simulink model "ex5_RL"  (R2023a)
settings: Solver=VariableStepAuto  StartTime=0.0  StopTime=30  RelTol=1e-3
values from neighbouring files (symbols this model uses):
  k1 = 5    [ex3_4.m]    (also in ex5.m = 1)
  k2 = 5    [ex3_4.m]    (also in ex5.m = 2.5)
  k3 = 3    [ex5.m]
  theta_i = qi(3)    [ex3_4.m]    (also in ex5.m = 0.785398163397)
  Ts = Ts * scaling    [ex3_4.m]    (also in ex5.m = 0.001)
  x_i = qi(1)    [ex3_4.m]    (also in ex5.m = 10)
  y_i = qi(2)    [ex3_4.m]    (also in ex5.m = 1)
libraries: robotmobilelib x1
settings Model: Creator=Francesco  LastModifiedBy=salvatoregranata
settings DataIOCC: ExternalInput=k1,k2 ,3
settings OptimizationCC: ReuseModelBlockBuffer=off
settings HardwareCC: ProdBitPerLong=64  ProdHWDeviceType=Intel->x86-64 (Mac OS X)

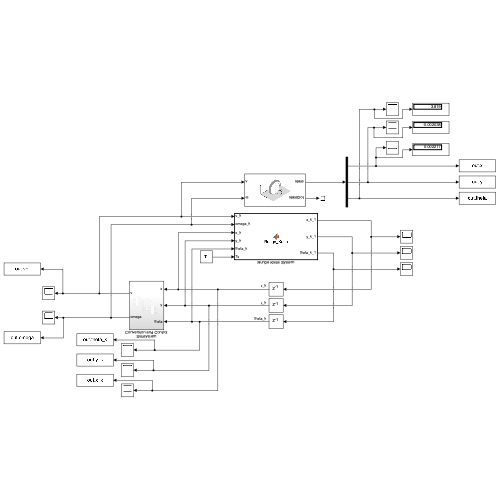
[thumbnail: Simulink's stored preview of the top-level diagram]
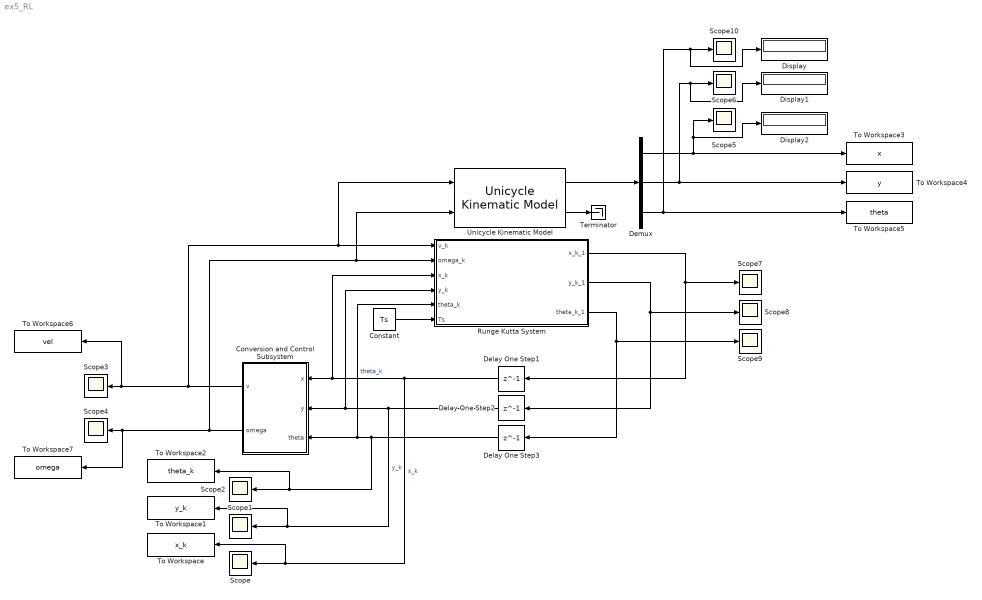
== system ex5_RL ==
  Constant : Constant  Value=Ts
  Conversion and Control Subsystem : Subsystem
  Delay One Step1 : Delay  DelayLength=1  InitialCondition=x_i  SampleTime=Ts
  Delay One Step2 : Delay  DelayLength=1  InitialCondition=y_i  SampleTime=Ts
  Delay One Step3 : Delay  DelayLength=1  InitialCondition=theta_i  SampleTime=Ts
  Demux : Demux  Outputs=3
  Display : Display
  Display1 : Display
  Display2 : Display
  Runge Kutta System : MATLAB Function  TreatAsAtomicUnit=on
  Scope{,1..10} (11 alike) : Scope
  Terminator : Terminator
  To Workspace : ToWorkspace  VariableName=x_k  SampleTime=-1
  To Workspace1 : ToWorkspace  VariableName=y_k  SampleTime=-1
  To Workspace2 : ToWorkspace  VariableName=theta_k  SampleTime=-1
  To Workspace3 : ToWorkspace  VariableName=x  SampleTime=-1
  To Workspace4 : ToWorkspace  VariableName=y  SampleTime=-1
  To Workspace5 : ToWorkspace  VariableName=theta  SaveFormat=Timeseries  SampleTime=-1
  To Workspace6 : ToWorkspace  VariableName=vel  SaveFormat=Timeseries  SampleTime=-1
  To Workspace7 : ToWorkspace  VariableName=omega  SaveFormat=Timeseries  SampleTime=-1
  Unicycle Kinematic Model : robotmobilelib/Unicycle Kinematic Model  VehicleInputs=Vehicle Speed & Heading Angular Velocity  WheelRadius=0.1  WheelSpeedRange=[-Inf Inf]  InitialState=[x_i; y_i; theta_i]  SimulateUsing=Interpreted execution
  wires:
  Runge Kutta System/3(theta_k_1) -> Delay One Step3/1, Scope9/1
  Delay One Step1/1 -> Runge Kutta System/3(x_k), Conversion and Control Subsystem/1(x), To Workspace/1, Scope/1  "x_k"
  Runge Kutta System/1(x_k_1) -> Scope7/1, Delay One Step1/1
  Delay One Step2/1 -> Runge Kutta System/4(y_k), Conversion and Control Subsystem/2(y), To Workspace1/1, Scope1/1  "y_k"
  Runge Kutta System/2(y_k_1) -> Delay One Step2/1, Scope8/1
  Unicycle Kinematic Model/1 -> Demux/1
  Demux/1 -> To Workspace3/1, Scope5/1, Display2/1
  Demux/2 -> To Workspace4/1, Display1/1, Scope6/1
  Delay One Step3/1 -> Conversion and Control Subsystem/3(theta), Runge Kutta System/5(theta_k), Scope2/1, To Workspace2/1  "theta_k"
  Conversion and Control Subsystem/1(v) -> Unicycle Kinematic Model/1, Runge Kutta System/1(v_k), To Workspace6/1, Scope3/1
  Conversion and Control Subsystem/2(omega) -> Unicycle Kinematic Model/2, Runge Kutta System/2(omega_k), To Workspace7/1, Scope4/1
  Demux/3 -> To Workspace5/1, Display/1, Scope10/1
  Unicycle Kinematic Model/2 -> Terminator/1
  Constant/1 -> Runge Kutta System/6(Ts)

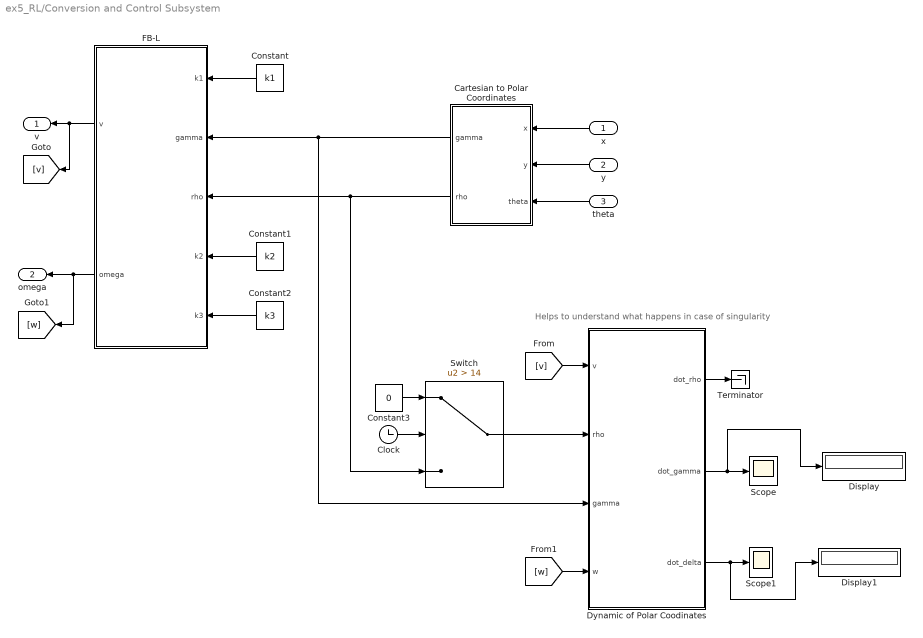
== system ex5_RL/Conversion and Control Subsystem ==
  note: Helps to understand what happens in case of singularity
  x : Inport
  y : Inport  Port=2
  theta : Inport  Port=3
  "Cartesian to Polar Coordinates " : Subsystem
  Clock : Clock
  Constant : Constant  Value=k1
  Constant1 : Constant  Value=k2
  Constant2 : Constant  Value=k3
  Constant3 : Constant  Value=0
  Display : Display
  Display1 : Display
  Dynamic of Polar Coodinates : MATLAB Function  TreatAsAtomicUnit=on
  FB-L : Subsystem
  Scope : Scope
  Scope1 : Scope
  Switch : Switch  Criteria=u2 > Threshold  Threshold=14  SaturateOnIntegerOverflow=off  InputSameDT=off
  Terminator : Terminator
  v : Outport
  omega : Outport  Port=2
  wires:
  Constant/1 -> FB-L/1(k1)
  Constant1/1 -> FB-L/4(k2)
  Constant2/1 -> FB-L/5(k3)
  FB-L/1(v) -> [v], v/1
  FB-L/2(omega) -> [w], omega/1
  x/1 -> "Cartesian to Polar Coordinates "/1(x)
  y/1 -> "Cartesian to Polar Coordinates "/2(y)
  theta/1 -> "Cartesian to Polar Coordinates "/3(theta)
  "Cartesian to Polar Coordinates "/2(rho) -> Switch/3, FB-L/3(rho)
  [v] -> Dynamic of Polar Coodinates/1(v)
  "Cartesian to Polar Coordinates "/1(gamma) -> Dynamic of Polar Coodinates/3(gamma), FB-L/2(gamma)
  [w] -> Dynamic of Polar Coodinates/4(w)
  Dynamic of Polar Coodinates/1(dot_rho) -> Terminator/1
  Dynamic of Polar Coodinates/2(dot_gamma) -> Display/1, Scope/1
  Dynamic of Polar Coodinates/3(dot_delta) -> Display1/1, Scope1/1
  Switch/1 -> Dynamic of Polar Coodinates/2(rho)
  Constant3/1 -> Switch/1
  Clock/1 -> Switch/2

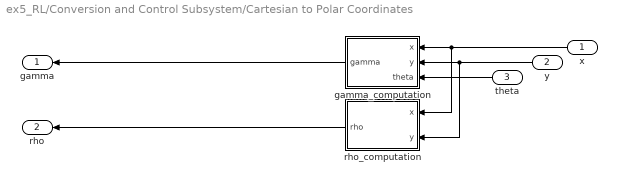
== system ex5_RL/Conversion and Control Subsystem/Cartesian to Polar Coordinates  ==
  x : Inport
  y : Inport  Port=2
  theta : Inport  Port=3
  gamma_computation : MATLAB Function  TreatAsAtomicUnit=on
  rho_computation : MATLAB Function  TreatAsAtomicUnit=on
  gamma : Outport
  rho : Outport  Port=2
  wires:
  gamma_computation/1(gamma) -> gamma/1
  theta/1 -> gamma_computation/3(theta)
  y/1 -> gamma_computation/2(y), rho_computation/2(y)
  rho_computation/1(rho) -> rho/1
  x/1 -> rho_computation/1(x), gamma_computation/1(x)

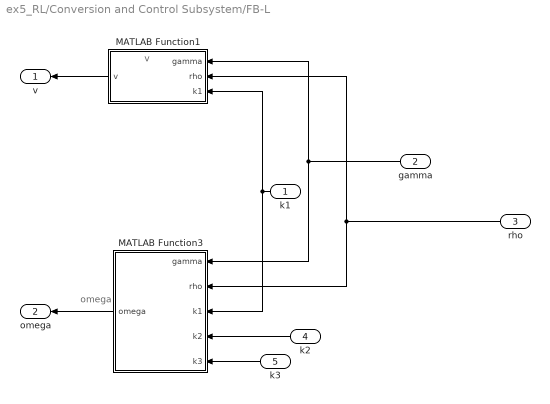
== system ex5_RL/Conversion and Control Subsystem/FB-L ==
  note: omega
  note: v
  k1 : Inport
  gamma : Inport  Port=2
  rho : Inport  Port=3
  k2 : Inport  Port=4
  k3 : Inport  Port=5
  MATLAB Function1 : MATLAB Function  TreatAsAtomicUnit=on
  MATLAB Function3 : MATLAB Function  TreatAsAtomicUnit=on
  v : Outport
  omega : Outport  Port=2
  wires:
  MATLAB Function1/1(v) -> v/1
  MATLAB Function3/1(omega) -> omega/1
  gamma/1 -> MATLAB Function1/1(gamma), MATLAB Function3/1(gamma)
  k1/1 -> MATLAB Function3/3(k1), MATLAB Function1/3(k1)
  k3/1 -> MATLAB Function3/5(k3)
  k2/1 -> MATLAB Function3/4(k2)
  rho/1 -> MATLAB Function3/2(rho), MATLAB Function1/2(rho)

== matlab function ex5_RL/Runge Kutta System ==
  data: v_k input; x_k_1 output; omega_k input; x_k input; y_k_1 output; y_k input; theta_k input; theta_k_1 output; Ts input
function [x_k_1,y_k_1,theta_k_1] = Runge_Kutta(v_k,omega_k,x_k,y_k,theta_k,Ts)

%2nd order Runge-Kutta approximation
x_k_1=x_k+v_k*Ts*cos(theta_k+Ts*omega_k/2);
y_k_1=y_k+v_k*Ts*sin(theta_k+Ts*omega_k/2);
theta_k_1=theta_k+omega_k*Ts;

== matlab function ex5_RL/Conversion and Control Subsystem/Cartesian to Polar Coordinates /rho_computation ==
  data: x input; rho output; y input
function rho = fcn(x,y)

rho=sqrt(x^2 + y^2);

== matlab function ex5_RL/Conversion and Control Subsystem/Cartesian to Polar Coordinates /gamma_computation ==
  data: x input; gamma output; y input; theta input
function gamma = fcn(x,y,theta)
gamma=atan2(y,x)-theta+pi;

== matlab function ex5_RL/Conversion and Control Subsystem/FB-L/MATLAB Function1 ==
  data: gamma input; rho input; v output; k1 input
function v = fcn(gamma,rho,k1)

v = k1*rho*cos(gamma);

== matlab function ex5_RL/Conversion and Control Subsystem/FB-L/MATLAB Function3 ==
  data: gamma input; omega output; rho input; k1 input; k2 input; k3 input
function omega = fcn(gamma,rho,k1,k2,k3)

delta=rho+gamma;

omega = k2*gamma+k1*sin(gamma)*cos(gamma)*(1+k3*(delta/gamma));

== matlab function ex5_RL/Conversion and Control Subsystem/Dynamic of Polar Coodinates ==
  data: v input; dot_rho output; rho input; gamma input; w input; dot_gamma output; dot_delta output
function [dot_rho,dot_gamma, dot_delta] = PolarDynamics(v,rho,gamma,w)
dot_rho=-v*cos(gamma);
dot_gamma=-sin(gamma)*v/rho - w;
dot_delta=sin(gamma)*v/rho;
